simulink model "servomotor_pi"  (R2020b)
settings: Solver=FixedStepAuto  StartTime=0.0  StopTime=tempoSimulacao  FixedStep=1e-4  RelTol=1e-3
values from neighbouring files (symbols this model uses):
  controlador = projetarControladorPI(planta, requisitos)    [avaliarIndutor.m]
  planta = obterPlantaServo()    [avaliarIndutor.m]
undefined symbols (not defined in the file or in its folder): disturbio, referencia
settings Model: Creator=mmaximo  LastModifiedBy=rudog

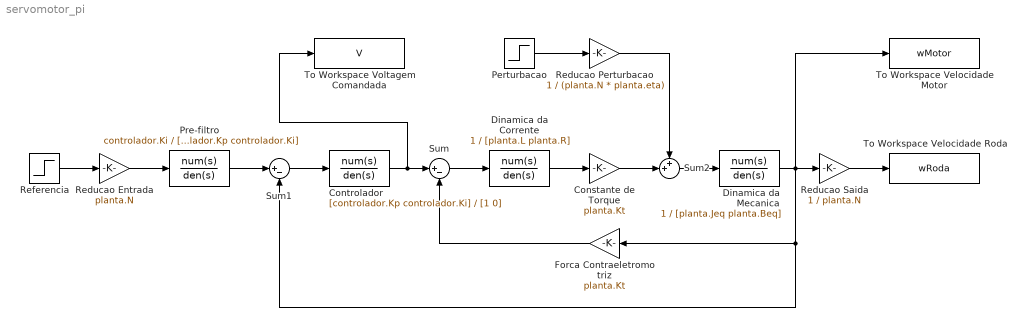
== system servomotor_pi ==
  Constante de Torque : Gain  Gain=planta.Kt
  Controlador : TransferFcn  Numerator=[controlador.Kp controlador.Ki]  Denominator=[1 0]
  Dinamica da Corrente : TransferFcn  Numerator=1  Denominator=[planta.L planta.R]
  Dinamica da Mecanica : TransferFcn  Numerator=1  Denominator=[planta.Jeq planta.Beq]
  Forca Contraeletromotriz : Gain  Gain=planta.Kt
  Perturbacao : Step  Time=disturbio.instante  After=disturbio.amplitude  SampleTime=0
  Pre-filtro : TransferFcn  Numerator=controlador.Ki  Denominator=[controlador.Kp controlador.Ki]
  Reducao Entrada : Gain  Gain=planta.N
  Reducao Perturbacao : Gain  Gain=1 / (planta.N * planta.eta)
  Reducao Saida : Gain  Gain=1 / planta.N
  Referencia : Step  Time=referencia.instante  After=referencia.amplitude  SampleTime=0
  Sum : Sum  Inputs=|+-
  Sum1 : Sum  Inputs=|+-
  Sum2 : Sum  Inputs=++|
  To Workspace Velocidade Motor : ToWorkspace  VariableName=wMotor  SaveFormat=Structure With Time  SampleTime=-1
  To Workspace Velocidade Roda : ToWorkspace  VariableName=wRoda  SaveFormat=Structure With Time  SampleTime=-1
  To Workspace Voltagem Comandada : ToWorkspace  VariableName=V  SaveFormat=Structure With Time  SampleTime=-1
  wires:
  Reducao Saida/1 -> To Workspace Velocidade Roda/1
  Referencia/1 -> Reducao Entrada/1
  Sum2/1 -> Dinamica da Mecanica/1
  Sum1/1 -> Controlador/1
  Dinamica da Mecanica/1 -> Reducao Saida/1, Sum1/2, Forca Contraeletromotriz/1, To Workspace Velocidade Motor/1
  Pre-filtro/1 -> Sum1/1
  Sum/1 -> Dinamica da Corrente/1
  Forca Contraeletromotriz/1 -> Sum/2
  Reducao Perturbacao/1 -> Sum2/1
  Perturbacao/1 -> Reducao Perturbacao/1
  Constante de Torque/1 -> Sum2/2
  Reducao Entrada/1 -> Pre-filtro/1
  Dinamica da Corrente/1 -> Constante de Torque/1
  Controlador/1 -> To Workspace Voltagem Comandada/1, Sum/1
